simulink model "BallBalancingwFb"  (R2025a)
settings: Solver=VariableStepAuto  StartTime=0.0  StopTime=10.0  RelTol=1e-3
values from neighbouring files (symbols this model uses):
  K1 = Ke_lqr(1)- Kp*C(1)    [Lab3_BallBalancing.m]
  K2 = Ke_lqr(2) - Kp*C(2)    [Lab3_BallBalancing.m]
  K3 = Ke_lqr(3) - Kp*C(3)    [Lab3_BallBalancing.m]
  K4 = Ke_lqr(4) - Kp*C(4)    [Lab3_BallBalancing.m]
  Kb = 0.028    [Lab3_BallBalancing.m]
  Ki = -Ke_lqr(5)    [Lab3_BallBalancing.m]
  Km = 1    [Lab3_BallBalancing.m]
  Kp = 1    [Lab3_BallBalancing.m]
  T0 = 0.057    [Lab3_BallBalancing.m]
  zeta = 0.59    [Lab3_BallBalancing.m]
settings Model: Creator=Admin  LastModifiedBy=Admin

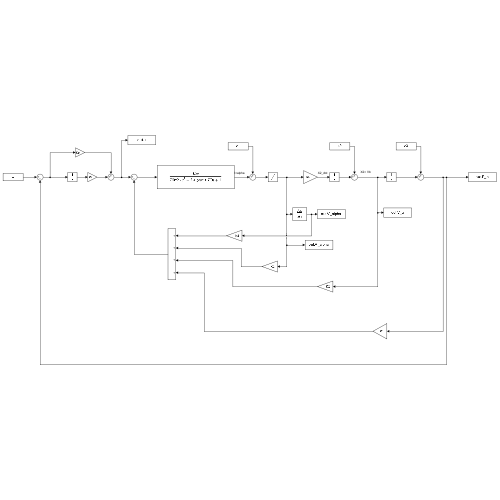
[thumbnail: Simulink's stored preview of the top-level diagram]
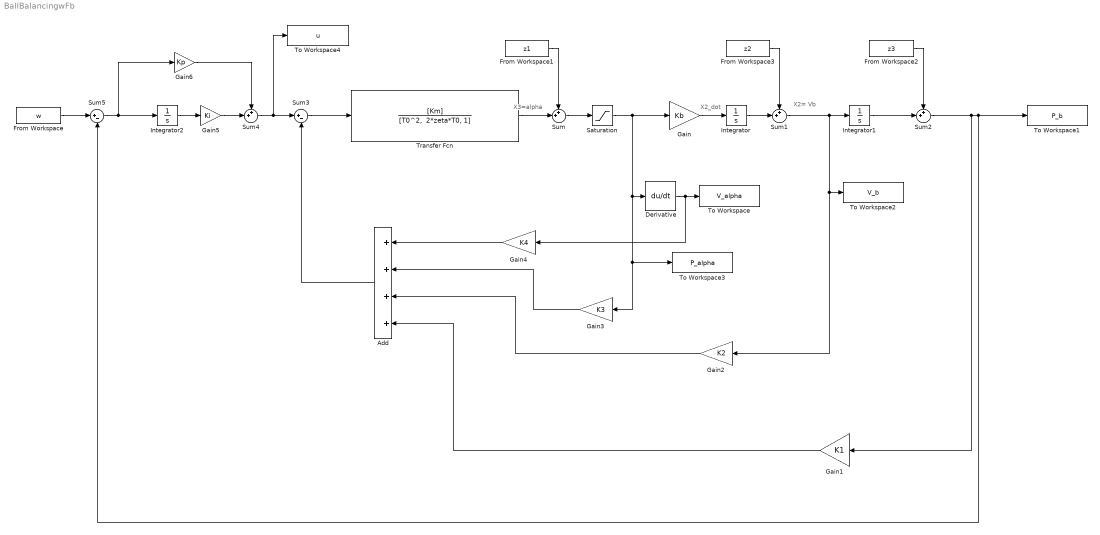
== system BallBalancingwFb ==
  note: X3=alpha
  note: X2_dot
  note: X2= Vb
  Add : Sum  Inputs=++++
  Derivative : Derivative
  From Workspace : FromWorkspace  VariableName=w
  From Workspace1 : FromWorkspace  VariableName=z1
  From Workspace2 : FromWorkspace  VariableName=z3
  From Workspace3 : FromWorkspace  VariableName=z2
  Gain : Gain  Gain=Kb
  Gain1 : Gain  Gain=K1
  Gain2 : Gain  Gain=K2
  Gain3 : Gain  Gain=K3
  Gain4 : Gain  Gain=K4
  Gain5 : Gain  Gain=Ki
  Gain6 : Gain  Gain=Kp
  Integrator : Integrator
  Integrator1 : Integrator
  Integrator2 : Integrator
  Saturation : Saturate  UpperLimit=45  LowerLimit=-45
  Sum{,1..2,4} (4 alike) : Sum  Inputs=++|
  Sum3 : Sum  Inputs=|+-
  Sum5 : Sum  Inputs=|+-
  To Workspace : ToWorkspace  VariableName=V_alpha  SaveFormat=Timeseries  SampleTime=-1
  To Workspace1 : ToWorkspace  VariableName=P_b  SaveFormat=Timeseries  SampleTime=-1
  To Workspace2 : ToWorkspace  VariableName=V_b  SaveFormat=Timeseries  SampleTime=-1
  To Workspace3 : ToWorkspace  VariableName=P_alpha  SaveFormat=Timeseries  SampleTime=-1
  To Workspace4 : ToWorkspace  VariableName=u  SaveFormat=Timeseries  SampleTime=-1
  Transfer Fcn : TransferFcn  Numerator=[Km]  Denominator="[T0^2,  2*zeta*T0, 1]"
  wires:
  Gain/1 -> Integrator/1
  Saturation/1 -> To Workspace3/1, Gain3/1, Derivative/1, Gain/1
  Derivative/1 -> Gain4/1, To Workspace/1
  Integrator1/1 -> Sum2/2
  Sum2/1 -> To Workspace1/1, Sum5/2, Gain1/1
  Integrator/1 -> Sum1/2
  Sum1/1 -> To Workspace2/1, Gain2/1, Integrator1/1
  From Workspace1/1 -> Sum/1
  Sum/1 -> Saturation/1
  Transfer Fcn/1 -> Sum/2
  From Workspace3/1 -> Sum1/1
  From Workspace2/1 -> Sum2/1
  Gain4/1 -> Add/1
  Gain3/1 -> Add/2
  Gain2/1 -> Add/3
  Gain1/1 -> Add/4
  Sum3/1 -> Transfer Fcn/1
  Add/1 -> Sum3/2
  Gain5/1 -> Sum4/2
  Sum4/1 -> To Workspace4/1, Sum3/1
  Gain6/1 -> Sum4/1
  Integrator2/1 -> Gain5/1
  Sum5/1 -> Gain6/1, Integrator2/1
  From Workspace/1 -> Sum5/1
